simulink model "qpsk"  (R2024a)
settings: Solver=VariableStepAuto  StartTime=0.0  StopTime=2e-3  RelTol=1e-3
libraries: dspsigops x20, simulink x2, commdigbbndpm3 x1, commrandsrc3 x1
(part 1 of 2)
settings Model: Creator=abc  LastModifiedBy=abc

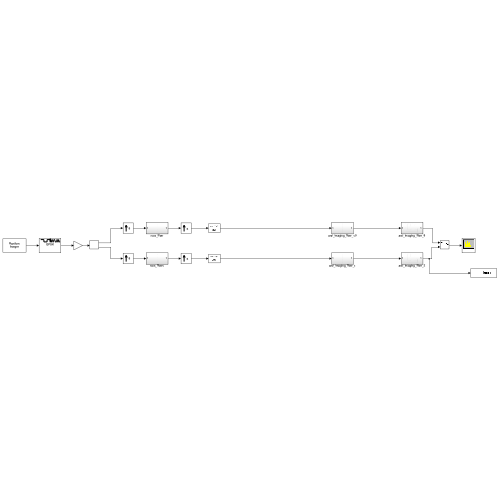
[thumbnail: Simulink's stored preview of the top-level diagram]
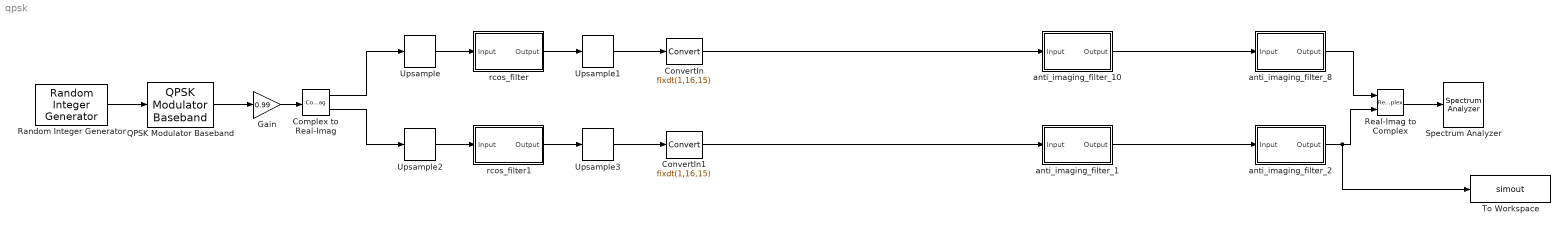
== system qpsk ==
  Complex to Real-Imag : ComplexToRealImag
  ConvertIn : DataTypeConversion  OutDataTypeStr=fixdt(1,16,15)  ConvertRealWorld=Stored Integer (SI)  RndMeth=Nearest
  ConvertIn1 : DataTypeConversion  OutDataTypeStr=fixdt(1,16,15)  ConvertRealWorld=Stored Integer (SI)  RndMeth=Nearest
  Gain : Gain  Gain=0.99
  QPSK Modulator Baseband : commdigbbndpm3/QPSK Modulator Baseband  InType=Integer  Enc=Gray  Ph=pi/4  outDtype=double  outWordLen=16  outUDDataType=sfix(16)  outFracLenMode=Best precision  outFracLen=15  outDataTypeStr=double  outLastDataTypeStr=double
  Random Integer Generator : commrandsrc3/Random Integer Generator  SetSize=4  SeedSource=Auto  Seed=0  SampleTime=1/(4.5e6)  SamplesPerFrame=1  OutputDataType=double  SimulateUsing=Interpreted execution
  Real-Imag to Complex : RealImagToComplex
  Spectrum Analyzer : SpectrumAnalyzer  WindowPosition=[56.000000,312.000000,800.000000,500.000000,]  ScopeFrameLocation=window  SampleRateSource=Property  SampleRate=1  Span=3600000.0000000005  StartFrequency=-1800000.0000000002  StopFrequency=1800000.0000000002  YLimits=[-27.09852792,27.05634095]  ExpandToolstrip=on
  To Workspace : ToWorkspace  VariableName=simout  SampleTime=-1
      settings: Save2DSignal=2-D array (concatenate along first dimension)
  Upsample : dspsigops/Upsample  FactorSource=Dialog parameter  N=8  Nmax=16  phase=0  InputProcessing=Columns as channels (frame based)  RateOptions=Allow multirate processing  ic=0  mode=Unused parameter value
  Upsample1 : dspsigops/Upsample  FactorSource=Dialog parameter  N=5  Nmax=16  phase=0  InputProcessing=Columns as channels (frame based)  RateOptions=Allow multirate processing  ic=0  mode=Unused parameter value
  Upsample2 : dspsigops/Upsample  FactorSource=Dialog parameter  N=8  Nmax=16  phase=0  InputProcessing=Columns as channels (frame based)  RateOptions=Allow multirate processing  ic=0  mode=Unused parameter value
  Upsample3 : dspsigops/Upsample  FactorSource=Dialog parameter  N=5  Nmax=16  phase=0  InputProcessing=Columns as channels (frame based)  RateOptions=Allow multirate processing  ic=0  mode=Unused parameter value
  anti_imaging_filter_1 : Subsystem  Tag=FilterWizardSubSystem
      settings: ErrorFcn=dspFilterRealizedInBasicElemsAlgLoopErrFcnCallback
  anti_imaging_filter_10 : Subsystem  Tag=FilterWizardSubSystem
      settings: ErrorFcn=dspFilterRealizedInBasicElemsAlgLoopErrFcnCallback
  anti_imaging_filter_2 : Subsystem  Tag=FilterWizardSubSystem
      settings: ErrorFcn=dspFilterRealizedInBasicElemsAlgLoopErrFcnCallback
  anti_imaging_filter_8 : Subsystem  Tag=FilterWizardSubSystem
      settings: ErrorFcn=dspFilterRealizedInBasicElemsAlgLoopErrFcnCallback
  rcos_filter : Subsystem  Tag=FilterWizardSubSystem
      settings: ErrorFcn=dspFilterRealizedInBasicElemsAlgLoopErrFcnCallback
  rcos_filter1 : Subsystem  Tag=FilterWizardSubSystem
      settings: ErrorFcn=dspFilterRealizedInBasicElemsAlgLoopErrFcnCallback
  wires:
  Random Integer Generator/1 -> QPSK Modulator Baseband/1
  QPSK Modulator Baseband/1 -> Gain/1
  Upsample/1 -> rcos_filter/1(Input)
  rcos_filter/1(Output) -> Upsample1/1
  Upsample1/1 -> ConvertIn/1
  anti_imaging_filter_10/1(Output) -> anti_imaging_filter_8/1(Input)
  ConvertIn/1 -> anti_imaging_filter_10/1(Input)
  Upsample2/1 -> rcos_filter1/1(Input)
  Upsample3/1 -> ConvertIn1/1
  rcos_filter1/1(Output) -> Upsample3/1
  ConvertIn1/1 -> anti_imaging_filter_1/1(Input)
  anti_imaging_filter_1/1(Output) -> anti_imaging_filter_2/1(Input)
  Gain/1 -> Complex to Real-Imag/1
  Complex to Real-Imag/1 -> Upsample/1
  Complex to Real-Imag/2 -> Upsample2/1
  anti_imaging_filter_8/1(Output) -> Real-Imag to Complex/1
  Real-Imag to Complex/1 -> Spectrum Analyzer/1
  anti_imaging_filter_2/1(Output) -> To Workspace/1, Real-Imag to Complex/2

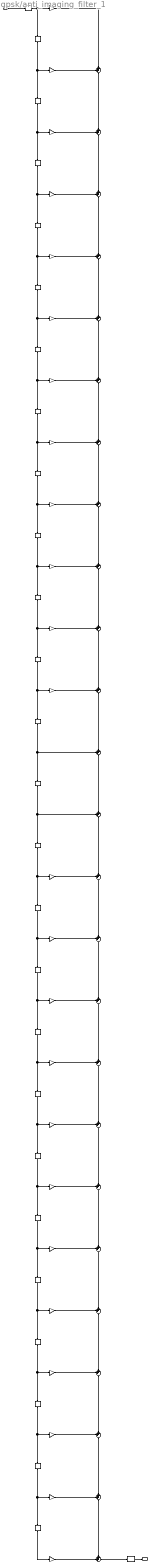
== system qpsk/anti_imaging_filter_1 ==
  Input : Inport
  BodyDelay{2..26} (25 alike) : Delay  DelayLength=1  InitialCondition=0  InputProcessing=Columns as channels (frame based)
  BodyLSum{2..26} (25 alike) : Sum  Inputs=++|  OutDataTypeStr=fixdt(1,35,30)  AccumDataTypeStr=fixdt(1,35,30)  RndMeth=Convergent
  ConvertIn : DataTypeConversion  OutDataTypeStr=fixdt(1,16,15)  RndMeth=Nearest
  ConvertOut : DataTypeConversion  OutDataTypeStr=fixdt(1,16,15)  RndMeth=Convergent  SaturateOnIntegerOverflow=off
  b(1) : Gain  Gain=0.0156626064233622506  ParamDataTypeStr=fixdt(1,16,15)  OutDataTypeStr=fixdt(1,31,30)  RndMeth=Convergent
  b(10) : Gain  Gain=0.784930628612014125  ParamDataTypeStr=fixdt(1,16,15)  OutDataTypeStr=fixdt(1,31,30)  RndMeth=Convergent
  b(11) : Gain  Gain=0.886772527356170293  ParamDataTypeStr=fixdt(1,16,15)  OutDataTypeStr=fixdt(1,31,30)  RndMeth=Convergent
  b(12) : Gain  Gain=0.960925295623340392  ParamDataTypeStr=fixdt(1,16,15)  OutDataTypeStr=fixdt(1,31,30)  RndMeth=Convergent
  b(15) : Gain  Gain=0.960925295623340392  ParamDataTypeStr=fixdt(1,16,15)  OutDataTypeStr=fixdt(1,31,30)  RndMeth=Convergent
  b(16) : Gain  Gain=0.886772527356170293  ParamDataTypeStr=fixdt(1,16,15)  OutDataTypeStr=fixdt(1,31,30)  RndMeth=Convergent
  b(17) : Gain  Gain=0.784930628612014125  ParamDataTypeStr=fixdt(1,16,15)  OutDataTypeStr=fixdt(1,31,30)  RndMeth=Convergent
  b(18) : Gain  Gain=0.665103266921935554  ParamDataTypeStr=fixdt(1,16,15)  OutDataTypeStr=fixdt(1,31,30)  RndMeth=Convergent
  b(19) : Gain  Gain=0.537919174813016099  ParamDataTypeStr=fixdt(1,16,15)  OutDataTypeStr=fixdt(1,31,30)  RndMeth=Convergent
  b(2) : Gain  Gain=0.0362761924333834043  ParamDataTypeStr=fixdt(1,16,15)  OutDataTypeStr=fixdt(1,31,30)  RndMeth=Convergent
  b(20) : Gain  Gain=0.413536705569194474  ParamDataTypeStr=fixdt(1,16,15)  OutDataTypeStr=fixdt(1,31,30)  RndMeth=Convergent
  b(21) : Gain  Gain=0.30040563304203749  ParamDataTypeStr=fixdt(1,16,15)  OutDataTypeStr=fixdt(1,31,30)  RndMeth=Convergent
  b(22) : Gain  Gain=0.204429372845306323  ParamDataTypeStr=fixdt(1,16,15)  OutDataTypeStr=fixdt(1,31,30)  RndMeth=Convergent
  b(23) : Gain  Gain=0.128628263180761093  ParamDataTypeStr=fixdt(1,16,15)  OutDataTypeStr=fixdt(1,31,30)  RndMeth=Convergent
  b(24) : Gain  Gain=0.0732387285445653402  ParamDataTypeStr=fixdt(1,16,15)  OutDataTypeStr=fixdt(1,31,30)  RndMeth=Convergent
  b(25) : Gain  Gain=0.0362761924333834043  ParamDataTypeStr=fixdt(1,16,15)  OutDataTypeStr=fixdt(1,31,30)  RndMeth=Convergent
  b(26) : Gain  Gain=0.0156626064233622506  ParamDataTypeStr=fixdt(1,16,15)  OutDataTypeStr=fixdt(1,31,30)  RndMeth=Convergent
  b(3) : Gain  Gain=0.0732387285445653402  ParamDataTypeStr=fixdt(1,16,15)  OutDataTypeStr=fixdt(1,31,30)  RndMeth=Convergent
  b(4) : Gain  Gain=0.128628263180761093  ParamDataTypeStr=fixdt(1,16,15)  OutDataTypeStr=fixdt(1,31,30)  RndMeth=Convergent
  b(5) : Gain  Gain=0.204429372845306323  ParamDataTypeStr=fixdt(1,16,15)  OutDataTypeStr=fixdt(1,31,30)  RndMeth=Convergent
  b(6) : Gain  Gain=0.30040563304203749  ParamDataTypeStr=fixdt(1,16,15)  OutDataTypeStr=fixdt(1,31,30)  RndMeth=Convergent
  b(7) : Gain  Gain=0.413536705569194474  ParamDataTypeStr=fixdt(1,16,15)  OutDataTypeStr=fixdt(1,31,30)  RndMeth=Convergent
  b(8) : Gain  Gain=0.537919174813016099  ParamDataTypeStr=fixdt(1,16,15)  OutDataTypeStr=fixdt(1,31,30)  RndMeth=Convergent
  b(9) : Gain  Gain=0.665103266921935554  ParamDataTypeStr=fixdt(1,16,15)  OutDataTypeStr=fixdt(1,31,30)  RndMeth=Convergent
  Output : Outport
  wires:
  Input/1 -> ConvertIn/1
  b(1)/1 -> BodyLSum2/2
  ConvertIn/1 -> b(1)/1, BodyDelay2/1
  BodyDelay2/1 -> b(2)/1, BodyDelay3/1
  b(2)/1 -> BodyLSum2/1
  BodyLSum2/1 -> BodyLSum3/2
  BodyDelay3/1 -> b(3)/1, BodyDelay4/1
  b(3)/1 -> BodyLSum3/1
  BodyLSum3/1 -> BodyLSum4/2
  BodyDelay4/1 -> b(4)/1, BodyDelay5/1
  b(4)/1 -> BodyLSum4/1
  BodyLSum4/1 -> BodyLSum5/2
  BodyDelay5/1 -> b(5)/1, BodyDelay6/1
  b(5)/1 -> BodyLSum5/1
  BodyLSum5/1 -> BodyLSum6/2
  BodyDelay6/1 -> b(6)/1, BodyDelay7/1
  b(6)/1 -> BodyLSum6/1
  BodyLSum6/1 -> BodyLSum7/2
  BodyDelay7/1 -> b(7)/1, BodyDelay8/1
  b(7)/1 -> BodyLSum7/1
  BodyLSum7/1 -> BodyLSum8/2
  BodyDelay8/1 -> b(8)/1, BodyDelay9/1
  b(8)/1 -> BodyLSum8/1
  BodyLSum8/1 -> BodyLSum9/2
  BodyDelay9/1 -> b(9)/1, BodyDelay10/1
  b(9)/1 -> BodyLSum9/1
  BodyLSum9/1 -> BodyLSum10/2
  BodyDelay10/1 -> b(10)/1, BodyDelay11/1
  b(10)/1 -> BodyLSum10/1
  BodyLSum10/1 -> BodyLSum11/2
  BodyDelay11/1 -> b(11)/1, BodyDelay12/1
  b(11)/1 -> BodyLSum11/1
  BodyLSum11/1 -> BodyLSum12/2
  BodyDelay12/1 -> b(12)/1, BodyDelay13/1
  b(12)/1 -> BodyLSum12/1
  BodyLSum12/1 -> BodyLSum13/2
  BodyDelay13/1 -> BodyLSum13/1, BodyDelay14/1
  BodyLSum13/1 -> BodyLSum14/2
  BodyDelay14/1 -> BodyLSum14/1, BodyDelay15/1
  BodyLSum14/1 -> BodyLSum15/2
  BodyDelay15/1 -> b(15)/1, BodyDelay16/1
  b(15)/1 -> BodyLSum15/1
  BodyLSum15/1 -> BodyLSum16/2
  BodyDelay16/1 -> b(16)/1, BodyDelay17/1
  b(16)/1 -> BodyLSum16/1
  BodyLSum16/1 -> BodyLSum17/2
  BodyDelay17/1 -> b(17)/1, BodyDelay18/1
  b(17)/1 -> BodyLSum17/1
  BodyLSum17/1 -> BodyLSum18/2
  BodyDelay18/1 -> b(18)/1, BodyDelay19/1
  b(18)/1 -> BodyLSum18/1
  BodyLSum18/1 -> BodyLSum19/2
  BodyDelay19/1 -> b(19)/1, BodyDelay20/1
  b(19)/1 -> BodyLSum19/1
  BodyLSum19/1 -> BodyLSum20/2
  BodyDelay20/1 -> b(20)/1, BodyDelay21/1
  b(20)/1 -> BodyLSum20/1
  BodyLSum20/1 -> BodyLSum21/2
  BodyDelay21/1 -> b(21)/1, BodyDelay22/1
  b(21)/1 -> BodyLSum21/1
  BodyLSum21/1 -> BodyLSum22/2
  BodyDelay22/1 -> b(22)/1, BodyDelay23/1
  b(22)/1 -> BodyLSum22/1
  BodyLSum22/1 -> BodyLSum23/2
  BodyDelay23/1 -> b(23)/1, BodyDelay24/1
  b(23)/1 -> BodyLSum23/1
  BodyLSum23/1 -> BodyLSum24/2
  BodyDelay24/1 -> b(24)/1, BodyDelay25/1
  b(24)/1 -> BodyLSum24/1
  BodyLSum24/1 -> BodyLSum25/2
  BodyDelay25/1 -> b(25)/1, BodyDelay26/1
  b(25)/1 -> BodyLSum25/1
  BodyLSum25/1 -> BodyLSum26/1
  BodyDelay26/1 -> b(26)/1
  b(26)/1 -> BodyLSum26/2
  BodyLSum26/1 -> ConvertOut/1
  ConvertOut/1 -> Output/1

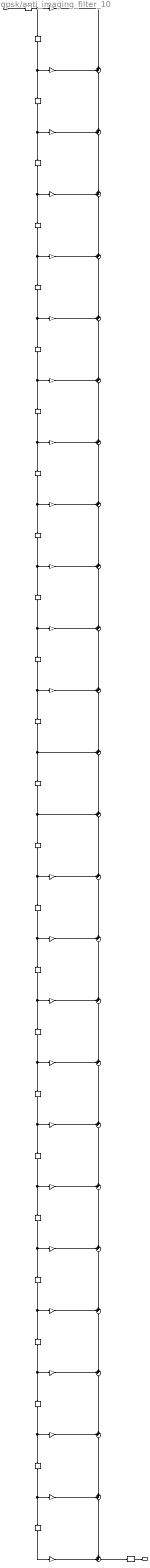
== system qpsk/anti_imaging_filter_10 ==
  Input : Inport
  BodyDelay{2..26} (25 alike) : Delay  DelayLength=1  InitialCondition=0  InputProcessing=Columns as channels (frame based)
  BodyLSum{2..26} (25 alike) : Sum  Inputs=++|  OutDataTypeStr=fixdt(1,35,30)  AccumDataTypeStr=fixdt(1,35,30)  RndMeth=Convergent
  ConvertIn : DataTypeConversion  OutDataTypeStr=fixdt(1,16,15)  RndMeth=Nearest
  ConvertOut : DataTypeConversion  OutDataTypeStr=fixdt(1,16,15)  RndMeth=Convergent  SaturateOnIntegerOverflow=off
  b(1) : Gain  Gain=0.0156626064233622506  ParamDataTypeStr=fixdt(1,16,15)  OutDataTypeStr=fixdt(1,31,30)  RndMeth=Convergent
  b(10) : Gain  Gain=0.784930628612014125  ParamDataTypeStr=fixdt(1,16,15)  OutDataTypeStr=fixdt(1,31,30)  RndMeth=Convergent
  b(11) : Gain  Gain=0.886772527356170293  ParamDataTypeStr=fixdt(1,16,15)  OutDataTypeStr=fixdt(1,31,30)  RndMeth=Convergent
  b(12) : Gain  Gain=0.960925295623340392  ParamDataTypeStr=fixdt(1,16,15)  OutDataTypeStr=fixdt(1,31,30)  RndMeth=Convergent
  b(15) : Gain  Gain=0.960925295623340392  ParamDataTypeStr=fixdt(1,16,15)  OutDataTypeStr=fixdt(1,31,30)  RndMeth=Convergent
  b(16) : Gain  Gain=0.886772527356170293  ParamDataTypeStr=fixdt(1,16,15)  OutDataTypeStr=fixdt(1,31,30)  RndMeth=Convergent
  b(17) : Gain  Gain=0.784930628612014125  ParamDataTypeStr=fixdt(1,16,15)  OutDataTypeStr=fixdt(1,31,30)  RndMeth=Convergent
  b(18) : Gain  Gain=0.665103266921935554  ParamDataTypeStr=fixdt(1,16,15)  OutDataTypeStr=fixdt(1,31,30)  RndMeth=Convergent
  b(19) : Gain  Gain=0.537919174813016099  ParamDataTypeStr=fixdt(1,16,15)  OutDataTypeStr=fixdt(1,31,30)  RndMeth=Convergent
  b(2) : Gain  Gain=0.0362761924333834043  ParamDataTypeStr=fixdt(1,16,15)  OutDataTypeStr=fixdt(1,31,30)  RndMeth=Convergent
  b(20) : Gain  Gain=0.413536705569194474  ParamDataTypeStr=fixdt(1,16,15)  OutDataTypeStr=fixdt(1,31,30)  RndMeth=Convergent
  b(21) : Gain  Gain=0.30040563304203749  ParamDataTypeStr=fixdt(1,16,15)  OutDataTypeStr=fixdt(1,31,30)  RndMeth=Convergent
  b(22) : Gain  Gain=0.204429372845306323  ParamDataTypeStr=fixdt(1,16,15)  OutDataTypeStr=fixdt(1,31,30)  RndMeth=Convergent
  b(23) : Gain  Gain=0.128628263180761093  ParamDataTypeStr=fixdt(1,16,15)  OutDataTypeStr=fixdt(1,31,30)  RndMeth=Convergent
  b(24) : Gain  Gain=0.0732387285445653402  ParamDataTypeStr=fixdt(1,16,15)  OutDataTypeStr=fixdt(1,31,30)  RndMeth=Convergent
  b(25) : Gain  Gain=0.0362761924333834043  ParamDataTypeStr=fixdt(1,16,15)  OutDataTypeStr=fixdt(1,31,30)  RndMeth=Convergent
  b(26) : Gain  Gain=0.0156626064233622506  ParamDataTypeStr=fixdt(1,16,15)  OutDataTypeStr=fixdt(1,31,30)  RndMeth=Convergent
  b(3) : Gain  Gain=0.0732387285445653402  ParamDataTypeStr=fixdt(1,16,15)  OutDataTypeStr=fixdt(1,31,30)  RndMeth=Convergent
  b(4) : Gain  Gain=0.128628263180761093  ParamDataTypeStr=fixdt(1,16,15)  OutDataTypeStr=fixdt(1,31,30)  RndMeth=Convergent
  b(5) : Gain  Gain=0.204429372845306323  ParamDataTypeStr=fixdt(1,16,15)  OutDataTypeStr=fixdt(1,31,30)  RndMeth=Convergent
  b(6) : Gain  Gain=0.30040563304203749  ParamDataTypeStr=fixdt(1,16,15)  OutDataTypeStr=fixdt(1,31,30)  RndMeth=Convergent
  b(7) : Gain  Gain=0.413536705569194474  ParamDataTypeStr=fixdt(1,16,15)  OutDataTypeStr=fixdt(1,31,30)  RndMeth=Convergent
  b(8) : Gain  Gain=0.537919174813016099  ParamDataTypeStr=fixdt(1,16,15)  OutDataTypeStr=fixdt(1,31,30)  RndMeth=Convergent
  b(9) : Gain  Gain=0.665103266921935554  ParamDataTypeStr=fixdt(1,16,15)  OutDataTypeStr=fixdt(1,31,30)  RndMeth=Convergent
  Output : Outport
  wires:
  Input/1 -> ConvertIn/1
  b(1)/1 -> BodyLSum2/2
  ConvertIn/1 -> b(1)/1, BodyDelay2/1
  BodyDelay2/1 -> b(2)/1, BodyDelay3/1
  b(2)/1 -> BodyLSum2/1
  BodyLSum2/1 -> BodyLSum3/2
  BodyDelay3/1 -> b(3)/1, BodyDelay4/1
  b(3)/1 -> BodyLSum3/1
  BodyLSum3/1 -> BodyLSum4/2
  BodyDelay4/1 -> b(4)/1, BodyDelay5/1
  b(4)/1 -> BodyLSum4/1
  BodyLSum4/1 -> BodyLSum5/2
  BodyDelay5/1 -> b(5)/1, BodyDelay6/1
  b(5)/1 -> BodyLSum5/1
  BodyLSum5/1 -> BodyLSum6/2
  BodyDelay6/1 -> b(6)/1, BodyDelay7/1
  b(6)/1 -> BodyLSum6/1
  BodyLSum6/1 -> BodyLSum7/2
  BodyDelay7/1 -> b(7)/1, BodyDelay8/1
  b(7)/1 -> BodyLSum7/1
  BodyLSum7/1 -> BodyLSum8/2
  BodyDelay8/1 -> b(8)/1, BodyDelay9/1
  b(8)/1 -> BodyLSum8/1
  BodyLSum8/1 -> BodyLSum9/2
  BodyDelay9/1 -> b(9)/1, BodyDelay10/1
  b(9)/1 -> BodyLSum9/1
  BodyLSum9/1 -> BodyLSum10/2
  BodyDelay10/1 -> b(10)/1, BodyDelay11/1
  b(10)/1 -> BodyLSum10/1
  BodyLSum10/1 -> BodyLSum11/2
  BodyDelay11/1 -> b(11)/1, BodyDelay12/1
  b(11)/1 -> BodyLSum11/1
  BodyLSum11/1 -> BodyLSum12/2
  BodyDelay12/1 -> b(12)/1, BodyDelay13/1
  b(12)/1 -> BodyLSum12/1
  BodyLSum12/1 -> BodyLSum13/2
  BodyDelay13/1 -> BodyLSum13/1, BodyDelay14/1
  BodyLSum13/1 -> BodyLSum14/2
  BodyDelay14/1 -> BodyLSum14/1, BodyDelay15/1
  BodyLSum14/1 -> BodyLSum15/2
  BodyDelay15/1 -> b(15)/1, BodyDelay16/1
  b(15)/1 -> BodyLSum15/1
  BodyLSum15/1 -> BodyLSum16/2
  BodyDelay16/1 -> b(16)/1, BodyDelay17/1
  b(16)/1 -> BodyLSum16/1
  BodyLSum16/1 -> BodyLSum17/2
  BodyDelay17/1 -> b(17)/1, BodyDelay18/1
  b(17)/1 -> BodyLSum17/1
  BodyLSum17/1 -> BodyLSum18/2
  BodyDelay18/1 -> b(18)/1, BodyDelay19/1
  b(18)/1 -> BodyLSum18/1
  BodyLSum18/1 -> BodyLSum19/2
  BodyDelay19/1 -> b(19)/1, BodyDelay20/1
  b(19)/1 -> BodyLSum19/1
  BodyLSum19/1 -> BodyLSum20/2
  BodyDelay20/1 -> b(20)/1, BodyDelay21/1
  b(20)/1 -> BodyLSum20/1
  BodyLSum20/1 -> BodyLSum21/2
  BodyDelay21/1 -> b(21)/1, BodyDelay22/1
  b(21)/1 -> BodyLSum21/1
  BodyLSum21/1 -> BodyLSum22/2
  BodyDelay22/1 -> b(22)/1, BodyDelay23/1
  b(22)/1 -> BodyLSum22/1
  BodyLSum22/1 -> BodyLSum23/2
  BodyDelay23/1 -> b(23)/1, BodyDelay24/1
  b(23)/1 -> BodyLSum23/1
  BodyLSum23/1 -> BodyLSum24/2
  BodyDelay24/1 -> b(24)/1, BodyDelay25/1
  b(24)/1 -> BodyLSum24/1
  BodyLSum24/1 -> BodyLSum25/2
  BodyDelay25/1 -> b(25)/1, BodyDelay26/1
  b(25)/1 -> BodyLSum25/1
  BodyLSum25/1 -> BodyLSum26/1
  BodyDelay26/1 -> b(26)/1
  b(26)/1 -> BodyLSum26/2
  BodyLSum26/1 -> ConvertOut/1
  ConvertOut/1 -> Output/1

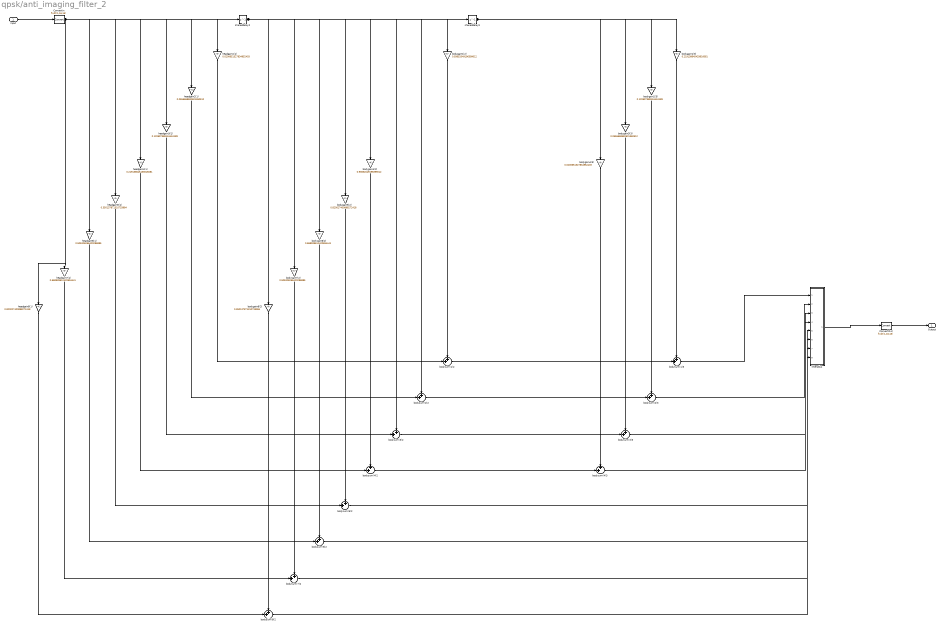
== system qpsk/anti_imaging_filter_2 ==
  Input : Inport
  ConvertIn : DataTypeConversion  OutDataTypeStr=fixdt(1,16,15)  RndMeth=Nearest
  ConvertOut : DataTypeConversion  OutDataTypeStr=fixdt(1,16,15)  RndMeth=Convergent  SaturateOnIntegerOverflow=off
  InterpSys : Subsystem  Tag=FilterWizardInterpolatorCommutator
  bodygain1(2) : Gain  Gain=0.93652049196399012  ParamDataTypeStr=fixdt(1,16,15)  OutDataTypeStr=fixdt(1,31,30)  RndMeth=Convergent
  bodygain1(3) : Gain  Gain=0.219138645433616081  ParamDataTypeStr=fixdt(1,16,15)  OutDataTypeStr=fixdt(1,31,30)  RndMeth=Convergent
  bodygain2(3) : Gain  Gain=0.120697388134434189  ParamDataTypeStr=fixdt(1,16,15)  OutDataTypeStr=fixdt(1,31,30)  RndMeth=Convergent
  bodygain3(3) : Gain  Gain=0.0556668582601360512  ParamDataTypeStr=fixdt(1,16,15)  OutDataTypeStr=fixdt(1,31,30)  RndMeth=Convergent
  bodygain4(2) : Gain  Gain=0.93652049196399012  ParamDataTypeStr=fixdt(1,16,15)  OutDataTypeStr=fixdt(1,31,30)  RndMeth=Convergent
  bodygain4(3) : Gain  Gain=0.0200651327834952403  ParamDataTypeStr=fixdt(1,16,15)  OutDataTypeStr=fixdt(1,31,30)  RndMeth=Convergent
  bodygain5(2) : Gain  Gain=0.820027400898272418  ParamDataTypeStr=fixdt(1,16,15)  OutDataTypeStr=fixdt(1,31,30)  RndMeth=Convergent
  bodygain6(2) : Gain  Gain=0.668939612420694441  ParamDataTypeStr=fixdt(1,16,15)  OutDataTypeStr=fixdt(1,31,30)  RndMeth=Convergent
  bodygain7(2) : Gain  Gain=0.505326266420286885  ParamDataTypeStr=fixdt(1,16,15)  OutDataTypeStr=fixdt(1,31,30)  RndMeth=Convergent
  bodygain8(2) : Gain  Gain=0.350137871310733984  ParamDataTypeStr=fixdt(1,16,15)  OutDataTypeStr=fixdt(1,31,30)  RndMeth=Convergent
  bodysum(1)2 : Sum  Inputs=++|  OutDataTypeStr=fixdt(1,35,30)  AccumDataTypeStr=fixdt(1,32,30)  RndMeth=Convergent
  bodysum(1)3 : Sum  Inputs=++|  OutDataTypeStr=fixdt(1,35,30)  AccumDataTypeStr=fixdt(1,32,30)  RndMeth=Convergent
  bodysum(2)2 : Sum  Inputs=++|  OutDataTypeStr=fixdt(1,35,30)  AccumDataTypeStr=fixdt(1,32,30)  RndMeth=Convergent
  bodysum(2)3 : Sum  Inputs=++|  OutDataTypeStr=fixdt(1,35,30)  AccumDataTypeStr=fixdt(1,32,30)  RndMeth=Convergent
  bodysum(3)2 : Sum  Inputs=++|  OutDataTypeStr=fixdt(1,35,30)  AccumDataTypeStr=fixdt(1,32,30)  RndMeth=Convergent
  bodysum(3)3 : Sum  Inputs=++|  OutDataTypeStr=fixdt(1,35,30)  AccumDataTypeStr=fixdt(1,32,30)  RndMeth=Convergent
  bodysum(4)2 : Sum  Inputs=++|  OutDataTypeStr=fixdt(1,35,30)  AccumDataTypeStr=fixdt(1,32,30)  RndMeth=Convergent
  bodysum(4)3 : Sum  Inputs=++|  OutDataTypeStr=fixdt(1,35,30)  AccumDataTypeStr=fixdt(1,32,30)  RndMeth=Convergent
  bodysum(5)2 : Sum  Inputs=++|  OutDataTypeStr=fixdt(1,35,30)  AccumDataTypeStr=fixdt(1,32,30)  RndMeth=Convergent
  bodysum(6)2 : Sum  Inputs=++|  OutDataTypeStr=fixdt(1,35,30)  AccumDataTypeStr=fixdt(1,32,30)  RndMeth=Convergent
  bodysum(7)2 : Sum  Inputs=++|  OutDataTypeStr=fixdt(1,35,30)  AccumDataTypeStr=fixdt(1,32,30)  RndMeth=Convergent
  bodysum(8)2 : Sum  Inputs=++|  OutDataTypeStr=fixdt(1,35,30)  AccumDataTypeStr=fixdt(1,32,30)  RndMeth=Convergent
  headgain1(1) : Gain  Gain=0.0200651327834952403  ParamDataTypeStr=fixdt(1,16,15)  OutDataTypeStr=fixdt(1,31,30)  RndMeth=Convergent
  headgain2(1) : Gain  Gain=0.0556668582601360512  ParamDataTypeStr=fixdt(1,16,15)  OutDataTypeStr=fixdt(1,31,30)  RndMeth=Convergent
  headgain3(1) : Gain  Gain=0.120697388134434189  ParamDataTypeStr=fixdt(1,16,15)  OutDataTypeStr=fixdt(1,31,30)  RndMeth=Convergent
  headgain4(1) : Gain  Gain=0.219138645433616081  ParamDataTypeStr=fixdt(1,16,15)  OutDataTypeStr=fixdt(1,31,30)  RndMeth=Convergent
  headgain5(1) : Gain  Gain=0.350137871310733984  ParamDataTypeStr=fixdt(1,16,15)  OutDataTypeStr=fixdt(1,31,30)  RndMeth=Convergent
  headgain6(1) : Gain  Gain=0.505326266420286885  ParamDataTypeStr=fixdt(1,16,15)  OutDataTypeStr=fixdt(1,31,30)  RndMeth=Convergent
  headgain7(1) : Gain  Gain=0.668939612420694441  ParamDataTypeStr=fixdt(1,16,15)  OutDataTypeStr=fixdt(1,31,30)  RndMeth=Convergent
  headgain8(1) : Gain  Gain=0.820027400898272418  ParamDataTypeStr=fixdt(1,16,15)  OutDataTypeStr=fixdt(1,31,30)  RndMeth=Convergent
  shareddelay2 : Delay  DelayLength=1  InitialCondition=0
  shareddelay3 : Delay  DelayLength=1  InitialCondition=0
  Output : Outport
  wires:
  headgain1(1)/1 -> bodysum(1)2/2
  headgain2(1)/1 -> bodysum(2)2/2
  headgain3(1)/1 -> bodysum(3)2/2
  headgain4(1)/1 -> bodysum(4)2/2
  headgain5(1)/1 -> bodysum(5)2/2
  headgain6(1)/1 -> bodysum(6)2/2
  headgain7(1)/1 -> bodysum(7)2/2
  headgain8(1)/1 -> bodysum(8)2/2
  Input/1 -> ConvertIn/1
  ConvertIn/1 -> headgain1(1)/1, headgain2(1)/1, headgain3(1)/1, headgain4(1)/1, headgain5(1)/1, headgain6(1)/1, headgain7(1)/1, headgain8(1)/1, shareddelay2/1
  bodygain1(2)/1 -> bodysum(1)2/1
  bodygain4(2)/1 -> bodysum(4)2/1
  bodygain5(2)/1 -> bodysum(5)2/1
  bodygain6(2)/1 -> bodysum(6)2/1
  bodygain7(2)/1 -> bodysum(7)2/1
  bodygain8(2)/1 -> bodysum(8)2/1
  bodysum(1)2/1 -> bodysum(1)3/2
  bodysum(2)2/1 -> bodysum(2)3/2
  bodysum(3)2/1 -> bodysum(3)3/2
  bodysum(4)2/1 -> bodysum(4)3/2
  bodysum(5)2/1 -> InterpSys/5(input5)
  bodysum(6)2/1 -> InterpSys/6(input6)
  bodysum(7)2/1 -> InterpSys/7(input7)
  bodysum(8)2/1 -> InterpSys/8(input8)
  shareddelay2/1 -> bodygain1(2)/1, bodysum(2)2/1, bodysum(3)2/1, bodygain4(2)/1, bodygain5(2)/1, bodygain6(2)/1, bodygain7(2)/1, bodygain8(2)/1, shareddelay3/1
  bodygain1(3)/1 -> bodysum(1)3/1
  bodygain2(3)/1 -> bodysum(2)3/1
  bodygain3(3)/1 -> bodysum(3)3/1
  bodygain4(3)/1 -> bodysum(4)3/1
  bodysum(1)3/1 -> InterpSys/1(input1)
  bodysum(2)3/1 -> InterpSys/2(input2)
  bodysum(3)3/1 -> InterpSys/3(input3)
  bodysum(4)3/1 -> InterpSys/4(input4)
  shareddelay3/1 -> bodygain1(3)/1, bodygain2(3)/1, bodygain3(3)/1, bodygain4(3)/1
  InterpSys/1(output) -> ConvertOut/1
  ConvertOut/1 -> Output/1

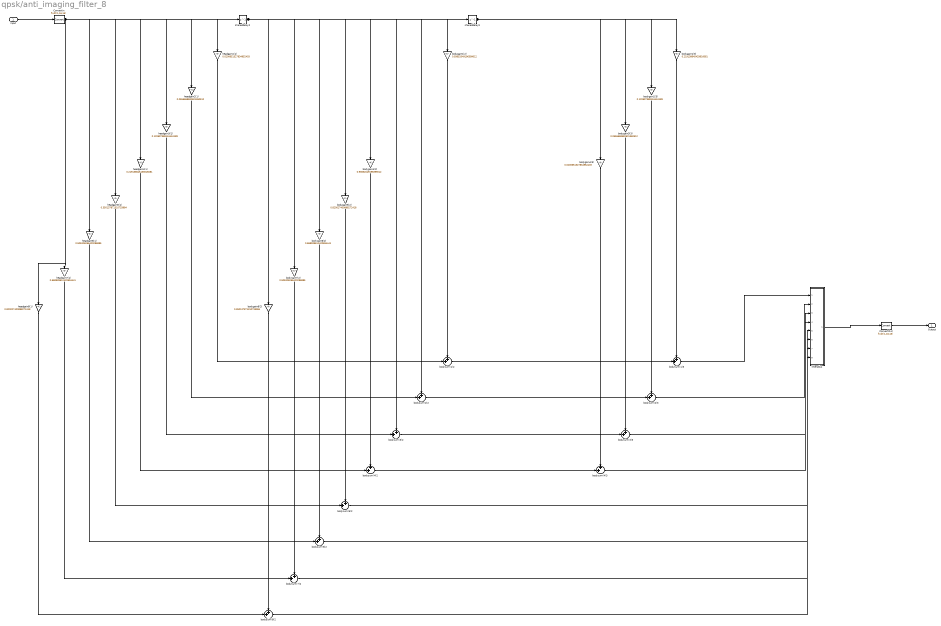
== system qpsk/anti_imaging_filter_8 ==
  Input : Inport
  ConvertIn : DataTypeConversion  OutDataTypeStr=fixdt(1,16,15)  RndMeth=Nearest
  ConvertOut : DataTypeConversion  OutDataTypeStr=fixdt(1,16,15)  RndMeth=Convergent  SaturateOnIntegerOverflow=off
  InterpSys : Subsystem  Tag=FilterWizardInterpolatorCommutator
  bodygain1(2) : Gain  Gain=0.93652049196399012  ParamDataTypeStr=fixdt(1,16,15)  OutDataTypeStr=fixdt(1,31,30)  RndMeth=Convergent
  bodygain1(3) : Gain  Gain=0.219138645433616081  ParamDataTypeStr=fixdt(1,16,15)  OutDataTypeStr=fixdt(1,31,30)  RndMeth=Convergent
  bodygain2(3) : Gain  Gain=0.120697388134434189  ParamDataTypeStr=fixdt(1,16,15)  OutDataTypeStr=fixdt(1,31,30)  RndMeth=Convergent
  bodygain3(3) : Gain  Gain=0.0556668582601360512  ParamDataTypeStr=fixdt(1,16,15)  OutDataTypeStr=fixdt(1,31,30)  RndMeth=Convergent
  bodygain4(2) : Gain  Gain=0.93652049196399012  ParamDataTypeStr=fixdt(1,16,15)  OutDataTypeStr=fixdt(1,31,30)  RndMeth=Convergent
  bodygain4(3) : Gain  Gain=0.0200651327834952403  ParamDataTypeStr=fixdt(1,16,15)  OutDataTypeStr=fixdt(1,31,30)  RndMeth=Convergent
  bodygain5(2) : Gain  Gain=0.820027400898272418  ParamDataTypeStr=fixdt(1,16,15)  OutDataTypeStr=fixdt(1,31,30)  RndMeth=Convergent
  bodygain6(2) : Gain  Gain=0.668939612420694441  ParamDataTypeStr=fixdt(1,16,15)  OutDataTypeStr=fixdt(1,31,30)  RndMeth=Convergent
  bodygain7(2) : Gain  Gain=0.505326266420286885  ParamDataTypeStr=fixdt(1,16,15)  OutDataTypeStr=fixdt(1,31,30)  RndMeth=Convergent
  bodygain8(2) : Gain  Gain=0.350137871310733984  ParamDataTypeStr=fixdt(1,16,15)  OutDataTypeStr=fixdt(1,31,30)  RndMeth=Convergent
  bodysum(1)2 : Sum  Inputs=++|  OutDataTypeStr=fixdt(1,35,30)  AccumDataTypeStr=fixdt(1,32,30)  RndMeth=Convergent
  bodysum(1)3 : Sum  Inputs=++|  OutDataTypeStr=fixdt(1,35,30)  AccumDataTypeStr=fixdt(1,32,30)  RndMeth=Convergent
  bodysum(2)2 : Sum  Inputs=++|  OutDataTypeStr=fixdt(1,35,30)  AccumDataTypeStr=fixdt(1,32,30)  RndMeth=Convergent
  bodysum(2)3 : Sum  Inputs=++|  OutDataTypeStr=fixdt(1,35,30)  AccumDataTypeStr=fixdt(1,32,30)  RndMeth=Convergent
  bodysum(3)2 : Sum  Inputs=++|  OutDataTypeStr=fixdt(1,35,30)  AccumDataTypeStr=fixdt(1,32,30)  RndMeth=Convergent
  bodysum(3)3 : Sum  Inputs=++|  OutDataTypeStr=fixdt(1,35,30)  AccumDataTypeStr=fixdt(1,32,30)  RndMeth=Convergent
  bodysum(4)2 : Sum  Inputs=++|  OutDataTypeStr=fixdt(1,35,30)  AccumDataTypeStr=fixdt(1,32,30)  RndMeth=Convergent
  bodysum(4)3 : Sum  Inputs=++|  OutDataTypeStr=fixdt(1,35,30)  AccumDataTypeStr=fixdt(1,32,30)  RndMeth=Convergent
  bodysum(5)2 : Sum  Inputs=++|  OutDataTypeStr=fixdt(1,35,30)  AccumDataTypeStr=fixdt(1,32,30)  RndMeth=Convergent
  bodysum(6)2 : Sum  Inputs=++|  OutDataTypeStr=fixdt(1,35,30)  AccumDataTypeStr=fixdt(1,32,30)  RndMeth=Convergent
  bodysum(7)2 : Sum  Inputs=++|  OutDataTypeStr=fixdt(1,35,30)  AccumDataTypeStr=fixdt(1,32,30)  RndMeth=Convergent
  bodysum(8)2 : Sum  Inputs=++|  OutDataTypeStr=fixdt(1,35,30)  AccumDataTypeStr=fixdt(1,32,30)  RndMeth=Convergent
  headgain1(1) : Gain  Gain=0.0200651327834952403  ParamDataTypeStr=fixdt(1,16,15)  OutDataTypeStr=fixdt(1,31,30)  RndMeth=Convergent
  headgain2(1) : Gain  Gain=0.0556668582601360512  ParamDataTypeStr=fixdt(1,16,15)  OutDataTypeStr=fixdt(1,31,30)  RndMeth=Convergent
  headgain3(1) : Gain  Gain=0.120697388134434189  ParamDataTypeStr=fixdt(1,16,15)  OutDataTypeStr=fixdt(1,31,30)  RndMeth=Convergent
  headgain4(1) : Gain  Gain=0.219138645433616081  ParamDataTypeStr=fixdt(1,16,15)  OutDataTypeStr=fixdt(1,31,30)  RndMeth=Convergent
  headgain5(1) : Gain  Gain=0.350137871310733984  ParamDataTypeStr=fixdt(1,16,15)  OutDataTypeStr=fixdt(1,31,30)  RndMeth=Convergent
  headgain6(1) : Gain  Gain=0.505326266420286885  ParamDataTypeStr=fixdt(1,16,15)  OutDataTypeStr=fixdt(1,31,30)  RndMeth=Convergent
  headgain7(1) : Gain  Gain=0.668939612420694441  ParamDataTypeStr=fixdt(1,16,15)  OutDataTypeStr=fixdt(1,31,30)  RndMeth=Convergent
  headgain8(1) : Gain  Gain=0.820027400898272418  ParamDataTypeStr=fixdt(1,16,15)  OutDataTypeStr=fixdt(1,31,30)  RndMeth=Convergent
  shareddelay2 : Delay  DelayLength=1  InitialCondition=0
  shareddelay3 : Delay  DelayLength=1  InitialCondition=0
  Output : Outport
  wires:
  headgain1(1)/1 -> bodysum(1)2/2
  headgain2(1)/1 -> bodysum(2)2/2
  headgain3(1)/1 -> bodysum(3)2/2
  headgain4(1)/1 -> bodysum(4)2/2
  headgain5(1)/1 -> bodysum(5)2/2
  headgain6(1)/1 -> bodysum(6)2/2
  headgain7(1)/1 -> bodysum(7)2/2
  headgain8(1)/1 -> bodysum(8)2/2
  Input/1 -> ConvertIn/1
  ConvertIn/1 -> headgain1(1)/1, headgain2(1)/1, headgain3(1)/1, headgain4(1)/1, headgain5(1)/1, headgain6(1)/1, headgain7(1)/1, headgain8(1)/1, shareddelay2/1
  bodygain1(2)/1 -> bodysum(1)2/1
  bodygain4(2)/1 -> bodysum(4)2/1
  bodygain5(2)/1 -> bodysum(5)2/1
  bodygain6(2)/1 -> bodysum(6)2/1
  bodygain7(2)/1 -> bodysum(7)2/1
  bodygain8(2)/1 -> bodysum(8)2/1
  bodysum(1)2/1 -> bodysum(1)3/2
  bodysum(2)2/1 -> bodysum(2)3/2
  bodysum(3)2/1 -> bodysum(3)3/2
  bodysum(4)2/1 -> bodysum(4)3/2
  bodysum(5)2/1 -> InterpSys/5(input5)
  bodysum(6)2/1 -> InterpSys/6(input6)
  bodysum(7)2/1 -> InterpSys/7(input7)
  bodysum(8)2/1 -> InterpSys/8(input8)
  shareddelay2/1 -> bodygain1(2)/1, bodysum(2)2/1, bodysum(3)2/1, bodygain4(2)/1, bodygain5(2)/1, bodygain6(2)/1, bodygain7(2)/1, bodygain8(2)/1, shareddelay3/1
  bodygain1(3)/1 -> bodysum(1)3/1
  bodygain2(3)/1 -> bodysum(2)3/1
  bodygain3(3)/1 -> bodysum(3)3/1
  bodygain4(3)/1 -> bodysum(4)3/1
  bodysum(1)3/1 -> InterpSys/1(input1)
  bodysum(2)3/1 -> InterpSys/2(input2)
  bodysum(3)3/1 -> InterpSys/3(input3)
  bodysum(4)3/1 -> InterpSys/4(input4)
  shareddelay3/1 -> bodygain1(3)/1, bodygain2(3)/1, bodygain3(3)/1, bodygain4(3)/1
  InterpSys/1(output) -> ConvertOut/1
  ConvertOut/1 -> Output/1

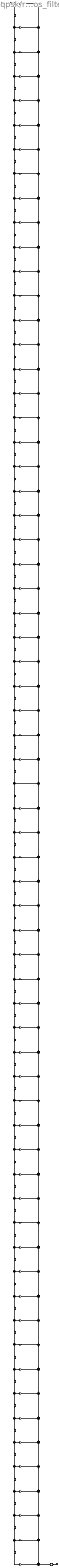
== system qpsk/rcos_filter ==
  Input : Inport
  BodyDelay{2..65} (64 alike) : Delay  DelayLength=1  InitialCondition=0  InputProcessing=Columns as channels (frame based)
  BodyLSum{2..65} (64 alike) : Sum  Inputs=++|  OutDataTypeStr=fixdt(1,35,30)  AccumDataTypeStr=fixdt(1,35,30)  RndMeth=Convergent
  ConvertIn : DataTypeConversion  OutDataTypeStr=fixdt(1,16,15)  RndMeth=Nearest
  ConvertOut : DataTypeConversion  OutDataTypeStr=fixdt(1,16,14)  RndMeth=Convergent  SaturateOnIntegerOverflow=off
  b(1) : Gain  Gain=-1.22182503891341904e-17  ParamDataTypeStr=fixdt(1,16,15)  OutDataTypeStr=fixdt(1,31,30)  RndMeth=Convergent
  b(10) : Gain  Gain=0.0244219543812943911  ParamDataTypeStr=fixdt(1,16,15)  OutDataTypeStr=fixdt(1,31,30)  RndMeth=Convergent
  b(11) : Gain  Gain=0.0496036323614192157  ParamDataTypeStr=fixdt(1,16,15)  OutDataTypeStr=fixdt(1,31,30)  RndMeth=Convergent
  b(12) : Gain  Gain=0.0711833868507990575  ParamDataTypeStr=fixdt(1,16,15)  OutDataTypeStr=fixdt(1,31,30)  RndMeth=Convergent
  b(13) : Gain  Gain=0.0845828249454869674  ParamDataTypeStr=fixdt(1,16,15)  OutDataTypeStr=fixdt(1,31,30)  RndMeth=Convergent
  b(14) : Gain  Gain=0.0857720064056135406  ParamDataTypeStr=fixdt(1,16,15)  OutDataTypeStr=fixdt(1,31,30)  RndMeth=Convergent
  b(15) : Gain  Gain=0.0720691236531740831  ParamDataTypeStr=fixdt(1,16,15)  OutDataTypeStr=fixdt(1,31,30)  RndMeth=Convergent
  b(16) : Gain  Gain=0.0428446671077597971  ParamDataTypeStr=fixdt(1,16,15)  OutDataTypeStr=fixdt(1,31,30)  RndMeth=Convergent
  b(17) : Gain  Gain=-3.01539353071549505e-17  ParamDataTypeStr=fixdt(1,16,15)  OutDataTypeStr=fixdt(1,31,30)  RndMeth=Convergent
  b(18) : Gain  Gain=-0.0518877257917480239  ParamDataTypeStr=fixdt(1,16,15)  OutDataTypeStr=fixdt(1,31,30)  RndMeth=Convergent
  b(19) : Gain  Gain=-0.105819956607615534  ParamDataTypeStr=fixdt(1,16,15)  OutDataTypeStr=fixdt(1,31,30)  RndMeth=Convergent
  b(2) : Gain  Gain=-0.0107228512436645974  ParamDataTypeStr=fixdt(1,16,15)  OutDataTypeStr=fixdt(1,31,30)  RndMeth=Convergent
  b(20) : Gain  Gain=-0.153038575384000536  ParamDataTypeStr=fixdt(1,16,15)  OutDataTypeStr=fixdt(1,31,30)  RndMeth=Convergent
  b(21) : Gain  Gain=-0.184039136773670148  ParamDataTypeStr=fixdt(1,16,15)  OutDataTypeStr=fixdt(1,31,30)  RndMeth=Convergent
  b(22) : Gain  Gain=-0.189818667042071343  ParamDataTypeStr=fixdt(1,16,15)  OutDataTypeStr=fixdt(1,31,30)  RndMeth=Convergent
  b(23) : Gain  Gain=-0.163194123759255266  ParamDataTypeStr=fixdt(1,16,15)  OutDataTypeStr=fixdt(1,31,30)  RndMeth=Convergent
  b(24) : Gain  Gain=-0.100002910003476192  ParamDataTypeStr=fixdt(1,16,15)  OutDataTypeStr=fixdt(1,31,30)  RndMeth=Convergent
  b(25) : Gain  Gain=3.66131944315138501e-17  ParamDataTypeStr=fixdt(1,16,15)  OutDataTypeStr=fixdt(1,31,30)  RndMeth=Convergent
  b(26) : Gain  Gain=0.132701532593299226  ParamDataTypeStr=fixdt(1,16,15)  OutDataTypeStr=fixdt(1,31,30)  RndMeth=Convergent
  b(27) : Gain  Gain=0.289741975985034095  ParamDataTypeStr=fixdt(1,16,15)  OutDataTypeStr=fixdt(1,31,30)  RndMeth=Convergent
  b(28) : Gain  Gain=0.459198248598821746  ParamDataTypeStr=fixdt(1,16,15)  OutDataTypeStr=fixdt(1,31,30)  RndMeth=Convergent
  b(29) : Gain  Gain=0.626776500752210253  ParamDataTypeStr=fixdt(1,16,15)  OutDataTypeStr=fixdt(1,31,30)  RndMeth=Convergent
  b(3) : Gain  Gain=-0.0221708270476338835  ParamDataTypeStr=fixdt(1,16,15)  OutDataTypeStr=fixdt(1,31,30)  RndMeth=Convergent
  b(30) : Gain  Gain=0.777375126299262864  ParamDataTypeStr=fixdt(1,16,15)  OutDataTypeStr=fixdt(1,31,30)  RndMeth=Convergent
  b(31) : Gain  Gain=0.896820714310533562  ParamDataTypeStr=fixdt(1,16,15)  OutDataTypeStr=fixdt(1,31,30)  RndMeth=Convergent
  b(32) : Gain  Gain=0.973548405003721196  ParamDataTypeStr=fixdt(1,16,15)  OutDataTypeStr=fixdt(1,31,30)  RndMeth=Convergent
  b(34) : Gain  Gain=0.973548405003721196  ParamDataTypeStr=fixdt(1,16,15)  OutDataTypeStr=fixdt(1,31,30)  RndMeth=Convergent
  b(35) : Gain  Gain=0.896820714310533562  ParamDataTypeStr=fixdt(1,16,15)  OutDataTypeStr=fixdt(1,31,30)  RndMeth=Convergent
  b(36) : Gain  Gain=0.777375126299262864  ParamDataTypeStr=fixdt(1,16,15)  OutDataTypeStr=fixdt(1,31,30)  RndMeth=Convergent
  b(37) : Gain  Gain=0.626776500752210253  ParamDataTypeStr=fixdt(1,16,15)  OutDataTypeStr=fixdt(1,31,30)  RndMeth=Convergent
  b(38) : Gain  Gain=0.459198248598821746  ParamDataTypeStr=fixdt(1,16,15)  OutDataTypeStr=fixdt(1,31,30)  RndMeth=Convergent
  b(39) : Gain  Gain=0.289741975985034095  ParamDataTypeStr=fixdt(1,16,15)  OutDataTypeStr=fixdt(1,31,30)  RndMeth=Convergent
  b(4) : Gain  Gain=-0.0323022715658651399  ParamDataTypeStr=fixdt(1,16,15)  OutDataTypeStr=fixdt(1,31,30)  RndMeth=Convergent
  b(40) : Gain  Gain=0.132701532593299226  ParamDataTypeStr=fixdt(1,16,15)  OutDataTypeStr=fixdt(1,31,30)  RndMeth=Convergent
  b(41) : Gain  Gain=3.66131944315138501e-17  ParamDataTypeStr=fixdt(1,16,15)  OutDataTypeStr=fixdt(1,31,30)  RndMeth=Convergent
  b(42) : Gain  Gain=-0.100002910003476192  ParamDataTypeStr=fixdt(1,16,15)  OutDataTypeStr=fixdt(1,31,30)  RndMeth=Convergent
  b(43) : Gain  Gain=-0.163194123759255266  ParamDataTypeStr=fixdt(1,16,15)  OutDataTypeStr=fixdt(1,31,30)  RndMeth=Convergent
  b(44) : Gain  Gain=-0.189818667042071343  ParamDataTypeStr=fixdt(1,16,15)  OutDataTypeStr=fixdt(1,31,30)  RndMeth=Convergent
  b(45) : Gain  Gain=-0.184039136773670148  ParamDataTypeStr=fixdt(1,16,15)  OutDataTypeStr=fixdt(1,31,30)  RndMeth=Convergent
  b(46) : Gain  Gain=-0.153038575384000536  ParamDataTypeStr=fixdt(1,16,15)  OutDataTypeStr=fixdt(1,31,30)  RndMeth=Convergent
  b(47) : Gain  Gain=-0.105819956607615534  ParamDataTypeStr=fixdt(1,16,15)  OutDataTypeStr=fixdt(1,31,30)  RndMeth=Convergent
  b(48) : Gain  Gain=-0.0518877257917480239  ParamDataTypeStr=fixdt(1,16,15)  OutDataTypeStr=fixdt(1,31,30)  RndMeth=Convergent
  b(49) : Gain  Gain=-3.01539353071549505e-17  ParamDataTypeStr=fixdt(1,16,15)  OutDataTypeStr=fixdt(1,31,30)  RndMeth=Convergent
  b(5) : Gain  Gain=-0.0388697150606156366  ParamDataTypeStr=fixdt(1,16,15)  OutDataTypeStr=fixdt(1,31,30)  RndMeth=Convergent
  b(50) : Gain  Gain=0.0428446671077597971  ParamDataTypeStr=fixdt(1,16,15)  OutDataTypeStr=fixdt(1,31,30)  RndMeth=Convergent
  b(51) : Gain  Gain=0.0720691236531740831  ParamDataTypeStr=fixdt(1,16,15)  OutDataTypeStr=fixdt(1,31,30)  RndMeth=Convergent
  b(52) : Gain  Gain=0.0857720064056135406  ParamDataTypeStr=fixdt(1,16,15)  OutDataTypeStr=fixdt(1,31,30)  RndMeth=Convergent
  b(53) : Gain  Gain=0.0845828249454869674  ParamDataTypeStr=fixdt(1,16,15)  OutDataTypeStr=fixdt(1,31,30)  RndMeth=Convergent
  b(54) : Gain  Gain=0.0711833868507990575  ParamDataTypeStr=fixdt(1,16,15)  OutDataTypeStr=fixdt(1,31,30)  RndMeth=Convergent
  b(55) : Gain  Gain=0.0496036323614192157  ParamDataTypeStr=fixdt(1,16,15)  OutDataTypeStr=fixdt(1,31,30)  RndMeth=Convergent
  b(56) : Gain  Gain=0.0244219543812943911  ParamDataTypeStr=fixdt(1,16,15)  OutDataTypeStr=fixdt(1,31,30)  RndMeth=Convergent
  b(57) : Gain  Gain=2.13059203422986562e-17  ParamDataTypeStr=fixdt(1,16,15)  OutDataTypeStr=fixdt(1,31,30)  RndMeth=Convergent
  b(58) : Gain  Gain=-0.0201382028340758128  ParamDataTypeStr=fixdt(1,16,15)  OutDataTypeStr=fixdt(1,31,30)  RndMeth=Convergent
  b(59) : Gain  Gain=-0.033708087527779762  ParamDataTypeStr=fixdt(1,16,15)  OutDataTypeStr=fixdt(1,31,30)  RndMeth=Convergent
  b(6) : Gain  Gain=-0.0398156990360692548  ParamDataTypeStr=fixdt(1,16,15)  OutDataTypeStr=fixdt(1,31,30)  RndMeth=Convergent
  b(60) : Gain  Gain=-0.0398156990360692548  ParamDataTypeStr=fixdt(1,16,15)  OutDataTypeStr=fixdt(1,31,30)  RndMeth=Convergent
  b(61) : Gain  Gain=-0.0388697150606156366  ParamDataTypeStr=fixdt(1,16,15)  OutDataTypeStr=fixdt(1,31,30)  RndMeth=Convergent
  b(62) : Gain  Gain=-0.0323022715658651399  ParamDataTypeStr=fixdt(1,16,15)  OutDataTypeStr=fixdt(1,31,30)  RndMeth=Convergent
  b(63) : Gain  Gain=-0.0221708270476338835  ParamDataTypeStr=fixdt(1,16,15)  OutDataTypeStr=fixdt(1,31,30)  RndMeth=Convergent
  b(64) : Gain  Gain=-0.0107228512436645974  ParamDataTypeStr=fixdt(1,16,15)  OutDataTypeStr=fixdt(1,31,30)  RndMeth=Convergent
  b(65) : Gain  Gain=-1.22182503891341904e-17  ParamDataTypeStr=fixdt(1,16,15)  OutDataTypeStr=fixdt(1,31,30)  RndMeth=Convergent
  b(7) : Gain  Gain=-0.033708087527779762  ParamDataTypeStr=fixdt(1,16,15)  OutDataTypeStr=fixdt(1,31,30)  RndMeth=Convergent
  b(8) : Gain  Gain=-0.0201382028340758128  ParamDataTypeStr=fixdt(1,16,15)  OutDataTypeStr=fixdt(1,31,30)  RndMeth=Convergent
  b(9) : Gain  Gain=2.13059203422986562e-17  ParamDataTypeStr=fixdt(1,16,15)  OutDataTypeStr=fixdt(1,31,30)  RndMeth=Convergent
  Output : Outport
  wires:
  Input/1 -> ConvertIn/1
  b(1)/1 -> BodyLSum2/2
  ConvertIn/1 -> b(1)/1, BodyDelay2/1
  BodyDelay2/1 -> b(2)/1, BodyDelay3/1
  b(2)/1 -> BodyLSum2/1
  BodyLSum2/1 -> BodyLSum3/2
  BodyDelay3/1 -> b(3)/1, BodyDelay4/1
  b(3)/1 -> BodyLSum3/1
  BodyLSum3/1 -> BodyLSum4/2
  BodyDelay4/1 -> b(4)/1, BodyDelay5/1
  b(4)/1 -> BodyLSum4/1
  BodyLSum4/1 -> BodyLSum5/2
  BodyDelay5/1 -> b(5)/1, BodyDelay6/1
  b(5)/1 -> BodyLSum5/1
  BodyLSum5/1 -> BodyLSum6/2
  BodyDelay6/1 -> b(6)/1, BodyDelay7/1
  b(6)/1 -> BodyLSum6/1
  BodyLSum6/1 -> BodyLSum7/2
  BodyDelay7/1 -> b(7)/1, BodyDelay8/1
  b(7)/1 -> BodyLSum7/1
  BodyLSum7/1 -> BodyLSum8/2
  BodyDelay8/1 -> b(8)/1, BodyDelay9/1
  b(8)/1 -> BodyLSum8/1
  BodyLSum8/1 -> BodyLSum9/2
  BodyDelay9/1 -> b(9)/1, BodyDelay10/1
  b(9)/1 -> BodyLSum9/1
  BodyLSum9/1 -> BodyLSum10/2
  BodyDelay10/1 -> b(10)/1, BodyDelay11/1
  b(10)/1 -> BodyLSum10/1
  BodyLSum10/1 -> BodyLSum11/2
  BodyDelay11/1 -> b(11)/1, BodyDelay12/1
  b(11)/1 -> BodyLSum11/1
  BodyLSum11/1 -> BodyLSum12/2
  BodyDelay12/1 -> b(12)/1, BodyDelay13/1
  b(12)/1 -> BodyLSum12/1
  BodyLSum12/1 -> BodyLSum13/2
  BodyDelay13/1 -> b(13)/1, BodyDelay14/1
  b(13)/1 -> BodyLSum13/1
  BodyLSum13/1 -> BodyLSum14/2
  BodyDelay14/1 -> b(14)/1, BodyDelay15/1
  b(14)/1 -> BodyLSum14/1
  BodyLSum14/1 -> BodyLSum15/2
  BodyDelay15/1 -> b(15)/1, BodyDelay16/1
  b(15)/1 -> BodyLSum15/1
  BodyLSum15/1 -> BodyLSum16/2
  BodyDelay16/1 -> b(16)/1, BodyDelay17/1
  b(16)/1 -> BodyLSum16/1
  BodyLSum16/1 -> BodyLSum17/2
  BodyDelay17/1 -> b(17)/1, BodyDelay18/1
  b(17)/1 -> BodyLSum17/1
  BodyLSum17/1 -> BodyLSum18/2
  BodyDelay18/1 -> b(18)/1, BodyDelay19/1
  b(18)/1 -> BodyLSum18/1
  BodyLSum18/1 -> BodyLSum19/2
  BodyDelay19/1 -> b(19)/1, BodyDelay20/1
  b(19)/1 -> BodyLSum19/1
  BodyLSum19/1 -> BodyLSum20/2
  BodyDelay20/1 -> b(20)/1, BodyDelay21/1
  b(20)/1 -> BodyLSum20/1
  BodyLSum20/1 -> BodyLSum21/2
  BodyDelay21/1 -> b(21)/1, BodyDelay22/1
  b(21)/1 -> BodyLSum21/1
  BodyLSum21/1 -> BodyLSum22/2
  BodyDelay22/1 -> b(22)/1, BodyDelay23/1
  b(22)/1 -> BodyLSum22/1
  BodyLSum22/1 -> BodyLSum23/2
  BodyDelay23/1 -> b(23)/1, BodyDelay24/1
  b(23)/1 -> BodyLSum23/1
  BodyLSum23/1 -> BodyLSum24/2
  BodyDelay24/1 -> b(24)/1, BodyDelay25/1
  b(24)/1 -> BodyLSum24/1
  BodyLSum24/1 -> BodyLSum25/2
  BodyDelay25/1 -> b(25)/1, BodyDelay26/1
  b(25)/1 -> BodyLSum25/1
  BodyLSum25/1 -> BodyLSum26/2
  BodyDelay26/1 -> b(26)/1, BodyDelay27/1
  b(26)/1 -> BodyLSum26/1
  BodyLSum26/1 -> BodyLSum27/2
  BodyDelay27/1 -> b(27)/1, BodyDelay28/1
  b(27)/1 -> BodyLSum27/1
  BodyLSum27/1 -> BodyLSum28/2
  BodyDelay28/1 -> b(28)/1, BodyDelay29/1
  b(28)/1 -> BodyLSum28/1
  BodyLSum28/1 -> BodyLSum29/2
  BodyDelay29/1 -> b(29)/1, BodyDelay30/1
  b(29)/1 -> BodyLSum29/1
  BodyLSum29/1 -> BodyLSum30/2
  BodyDelay30/1 -> b(30)/1, BodyDelay31/1
  b(30)/1 -> BodyLSum30/1
  BodyLSum30/1 -> BodyLSum31/2
  BodyDelay31/1 -> b(31)/1, BodyDelay32/1
  b(31)/1 -> BodyLSum31/1
  BodyLSum31/1 -> BodyLSum32/2
  BodyDelay32/1 -> b(32)/1, BodyDelay33/1
  b(32)/1 -> BodyLSum32/1
  BodyLSum32/1 -> BodyLSum33/2
  BodyDelay33/1 -> BodyLSum33/1, BodyDelay34/1
  BodyLSum33/1 -> BodyLSum34/2
  BodyDelay34/1 -> b(34)/1, BodyDelay35/1
  b(34)/1 -> BodyLSum34/1
  BodyLSum34/1 -> BodyLSum35/2
  BodyDelay35/1 -> b(35)/1, BodyDelay36/1
  b(35)/1 -> BodyLSum35/1
  BodyLSum35/1 -> BodyLSum36/2
  BodyDelay36/1 -> b(36)/1, BodyDelay37/1
  b(36)/1 -> BodyLSum36/1
  BodyLSum36/1 -> BodyLSum37/2
  BodyDelay37/1 -> b(37)/1, BodyDelay38/1
  b(37)/1 -> BodyLSum37/1
  BodyLSum37/1 -> BodyLSum38/2
  BodyDelay38/1 -> b(38)/1, BodyDelay39/1
  b(38)/1 -> BodyLSum38/1
  BodyLSum38/1 -> BodyLSum39/2
  BodyDelay39/1 -> b(39)/1, BodyDelay40/1
  b(39)/1 -> BodyLSum39/1
  BodyLSum39/1 -> BodyLSum40/2
  BodyDelay40/1 -> b(40)/1, BodyDelay41/1
  b(40)/1 -> BodyLSum40/1
  BodyLSum40/1 -> BodyLSum41/2
  BodyDelay41/1 -> b(41)/1, BodyDelay42/1
  b(41)/1 -> BodyLSum41/1
  BodyLSum41/1 -> BodyLSum42/2
  BodyDelay42/1 -> b(42)/1, BodyDelay43/1
  b(42)/1 -> BodyLSum42/1
  BodyLSum42/1 -> BodyLSum43/2
  BodyDelay43/1 -> b(43)/1, BodyDelay44/1
  b(43)/1 -> BodyLSum43/1
  BodyLSum43/1 -> BodyLSum44/2
  BodyDelay44/1 -> b(44)/1, BodyDelay45/1
  b(44)/1 -> BodyLSum44/1
  BodyLSum44/1 -> BodyLSum45/2
  BodyDelay45/1 -> b(45)/1, BodyDelay46/1
  b(45)/1 -> BodyLSum45/1
  BodyLSum45/1 -> BodyLSum46/2
  BodyDelay46/1 -> b(46)/1, BodyDelay47/1
  b(46)/1 -> BodyLSum46/1
  BodyLSum46/1 -> BodyLSum47/2
  BodyDelay47/1 -> b(47)/1, BodyDelay48/1
  b(47)/1 -> BodyLSum47/1
  BodyLSum47/1 -> BodyLSum48/2
  BodyDelay48/1 -> b(48)/1, BodyDelay49/1
  b(48)/1 -> BodyLSum48/1
  BodyLSum48/1 -> BodyLSum49/2
  BodyDelay49/1 -> b(49)/1, BodyDelay50/1
  b(49)/1 -> BodyLSum49/1
  BodyLSum49/1 -> BodyLSum50/2
  BodyDelay50/1 -> b(50)/1, BodyDelay51/1
  b(50)/1 -> BodyLSum50/1
  BodyLSum50/1 -> BodyLSum51/2
  BodyDelay51/1 -> b(51)/1, BodyDelay52/1
  b(51)/1 -> BodyLSum51/1
  BodyLSum51/1 -> BodyLSum52/2
  BodyDelay52/1 -> b(52)/1, BodyDelay53/1
  b(52)/1 -> BodyLSum52/1
  BodyLSum52/1 -> BodyLSum53/2
  BodyDelay53/1 -> b(53)/1, BodyDelay54/1
  b(53)/1 -> BodyLSum53/1
  BodyLSum53/1 -> BodyLSum54/2
  BodyDelay54/1 -> b(54)/1, BodyDelay55/1
  b(54)/1 -> BodyLSum54/1
  BodyLSum54/1 -> BodyLSum55/2
  BodyDelay55/1 -> b(55)/1, BodyDelay56/1
  b(55)/1 -> BodyLSum55/1
  BodyLSum55/1 -> BodyLSum56/2
  BodyDelay56/1 -> b(56)/1, BodyDelay57/1
  b(56)/1 -> BodyLSum56/1
  BodyLSum56/1 -> BodyLSum57/2
  BodyDelay57/1 -> b(57)/1, BodyDelay58/1
  b(57)/1 -> BodyLSum57/1
  BodyLSum57/1 -> BodyLSum58/2
  BodyDelay58/1 -> b(58)/1, BodyDelay59/1
  b(58)/1 -> BodyLSum58/1
  BodyLSum58/1 -> BodyLSum59/2
  BodyDelay59/1 -> b(59)/1, BodyDelay60/1
  b(59)/1 -> BodyLSum59/1
  BodyLSum59/1 -> BodyLSum60/2
  BodyDelay60/1 -> b(60)/1, BodyDelay61/1
  b(60)/1 -> BodyLSum60/1
  BodyLSum60/1 -> BodyLSum61/2
  BodyDelay61/1 -> b(61)/1, BodyDelay62/1
  b(61)/1 -> BodyLSum61/1
  BodyLSum61/1 -> BodyLSum62/2
  BodyDelay62/1 -> b(62)/1, BodyDelay63/1
  b(62)/1 -> BodyLSum62/1
  BodyLSum62/1 -> BodyLSum63/2
  BodyDelay63/1 -> b(63)/1, BodyDelay64/1
  b(63)/1 -> BodyLSum63/1
  BodyLSum63/1 -> BodyLSum64/2
  BodyDelay64/1 -> b(64)/1, BodyDelay65/1
  b(64)/1 -> BodyLSum64/1
  BodyLSum64/1 -> BodyLSum65/1
  BodyDelay65/1 -> b(65)/1
  b(65)/1 -> BodyLSum65/2
  BodyLSum65/1 -> ConvertOut/1
  ConvertOut/1 -> Output/1
